simulink model "ROM_draft2_5_sections"  (R2023a)
settings: Solver=ode15s  StartTime=0.0  StopTime=3  FixedStep=0.1  RelTol=1e-3
model workspace (MAT data in the model file):
  E_IVD4_N = 5
  E_IVD4_Z1 = 5
  E_IVD4_Z2 = 5
  E_IVD4_Z3 = 5
  E_IVD4_Z4 = 5
  E_IVD5_N = 5
  E_IVD5_Z1 = 5
  E_IVD5_Z2 = 5
  E_IVD5_Z3 = 5
  E_IVD5_Z4 = 5
  IVD4_N : object (value not decoded)
  IVD4_Z1 : object (value not decoded)
  IVD4_Z2 : object (value not decoded)
  IVD4_Z3 : object (value not decoded)
  IVD4_Z4 : object (value not decoded)
  IVD5_N : object (value not decoded)
  IVD5_Z1 : object (value not decoded)
  IVD5_Z2 : object (value not decoded)
  IVD5_Z3 : object (value not decoded)
  IVD5_Z4 : object (value not decoded)
  Moment_AR = 0
  Moment_FE = 0
  Moment_LB = 0
  ROM_draft1_sdosession : sldodialogs.data.SessionData (value not decoded)
  ROM_draft2_sdosession : sldodialogs.data.SessionData (value not decoded)
symbols that are objects in the model workspace (value not decoded): IVD4_N, IVD4_Z1, IVD4_Z2, IVD4_Z3, IVD4_Z4, IVD5_N, IVD5_Z1, IVD5_Z2, IVD5_Z3, IVD5_Z4
libraries: sm_lib x29, nesl_utility x9, checkpacklib x4, simulink_extras x4, simulink x1
(part 2 of 2)

== matlab function ROM_draft2_5_sections/MATLAB Function ==
  data: t input; FE output; LB output; AR output
function [FE, LB, AR] = switch_sine_wave(t)
%#codegen

% Define sine wave parameters for FE, LB, and AR
A_FE = 7.5; f_FE = 1;  % Amplitude and frequency for FE
A_LB = 7.5; f_LB = 1;  % Amplitude and frequency for LB
A_AR = 7.5; f_AR = 1;  % Amplitude and frequency for AR

% Initialize outputs to zero
FE = 0;
LB = 0;
AR = 0;

% Switch based on the simulation time
if t >= 0 && t < 1
    FE = A_FE * sin(2 * pi * f_FE * t);
    LB = 0;
    AR = 0;    
elseif t >= 1 && t < 2
    LB = A_LB * sin(2 * pi * f_LB * t);
    FE = 0;
    AR = 0;  
elseif t >= 2 && t <= 3
    AR = A_AR * sin(2 * pi * f_AR * t);
    FE = 0;
    LB = 0;
end
